simulink model "qpskrx_2022a"  (R2022a)
settings: Solver=FixedStepDiscrete  StartTime=0.0  StopTime=N*r/fs  RelTol=1e-3
values from neighbouring files (symbols this model uses):
  fs = oriFs*r    (= 750000000)    [LoadMat.m]    (also in test.m = 50000000; workspaceLoader.m = 75000000; workspaceLoader_fc32.m = 75000000; workspaceLoader_int16.m = 1500000000)
  rs = 75e6    (= 75000000)    [LoadMat.m]    (also in test.m = 37500000; workspaceLoader.m = 37500000; workspaceLoader_fc32.m = 37500000; workspaceLoader_int16.m)
libraries: commsync2 x2, commrfcorlib x1, dspsigops x1, commfilt2 x1
settings Model: FPTRunName=Active  Creator=The MathWorks, Inc.  LastModifiedBy=admin
settings SolverCC: AlgebraicLoopSolver=TrustRegion
settings DataIOCC: LimitDataPoints=on  SaveFormat=Structure  SaveOutput=off  SignalLogging=off  DSMLogging=off  SaveTime=off  ReturnWorkspaceOutputs=off
settings OptimizationCC: DefaultParameterBehavior=Inlined  ExpressionDepthLimit=2147483647  LocalBlockOutputs=off  ZeroExternalMemoryAtStartup=off  ZeroInternalMemoryAtStartup=off  InitFltsAndDblsToZero=on  LifeSpan=inf  SimCompilerOptimization=on
settings DebuggingCC: AlgebraicLoopMsg=error  UnderspecifiedInitializationDetection=Classic  MergeDetectMultiDrivingBlocksExec=none  SolverPrmCheckMsg=warning  SingleTaskRateTransMsg=error  ParameterPrecisionLossMsg=none  FcnCallInpInsideContextMsg=warning  UnconnectedInputMsg=warning  UnconnectedOutputMsg=warning  UnconnectedLineMsg=warning  AllowSymbolicDim=off  StateNameClashWarn=warning  SFUnexpectedBacktrackingDiag=warning  SFNoUnconditionalDefaultTransitionDiag=warning  SFExecutionAtInitializationDiag=none  ArithmeticOperatorsInVariantConditions=warning
settings HardwareCC: ProdBitPerPointer=32  ProdBitPerSizeT=32  ProdBitPerPtrDiffT=32  ProdLargestAtomicFloat=None  ProdIntDivRoundTo=Undefined  ProdEndianess=Unspecified  ProdWordSize=32  ProdLongLongMode=on  ProdHWDeviceType=32-bit Generic  TargetBitPerPointer=64  TargetBitPerSizeT=64  TargetBitPerPtrDiffT=64  TargetLongLongMode=on  TargetIntDivRoundTo=Zero  TargetEndianess=LittleEndian  TargetWordSize=64  TargetHWDeviceType=Generic->MATLAB Host Computer  ProdEqTarget=off
settings ModelReferenceCC: PropagateSignalLabelsOutOfModel=off
settings SFSimCC: SimUseLocalCustomCode=off  CustomCodeUndefinedFunction=UseInterfaceOnly  SimTargetLang=C++  GPUAcceleration=on  SimDLTargetLibrary=cudnn
settings RTWCC: RTWUseLocalCustomCode=off  TargetLang=C++  DLArmComputeVersion=19.05
settings RTWCC: CustomSourceCode=|
  | #include <stdio.h>
  | #include <stdlib.h>
settings CodeAppCC: StateflowObjectComments=on
settings GRTTargetCC: TargetLangStandard=C++11 (ISO)  CodeInterfacePackaging=C++ class
settings ConfigComp: CovMetricSettings=dw  CovSaveCumulativeToWorkspaceVar=on  CovSaveSingleToWorkspaceVar=on  CovExternalEMLEnable=off  CovSFcnEnable=off

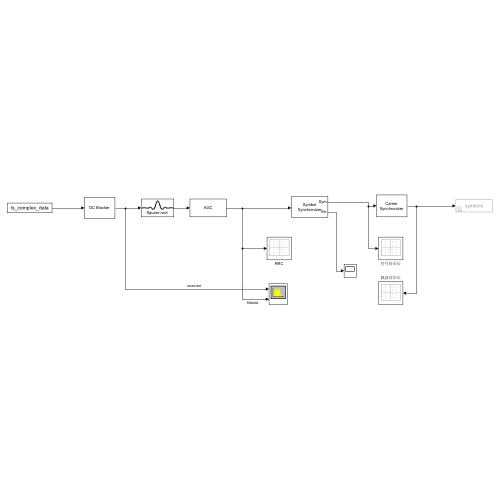
[thumbnail: Simulink's stored preview of the top-level diagram]
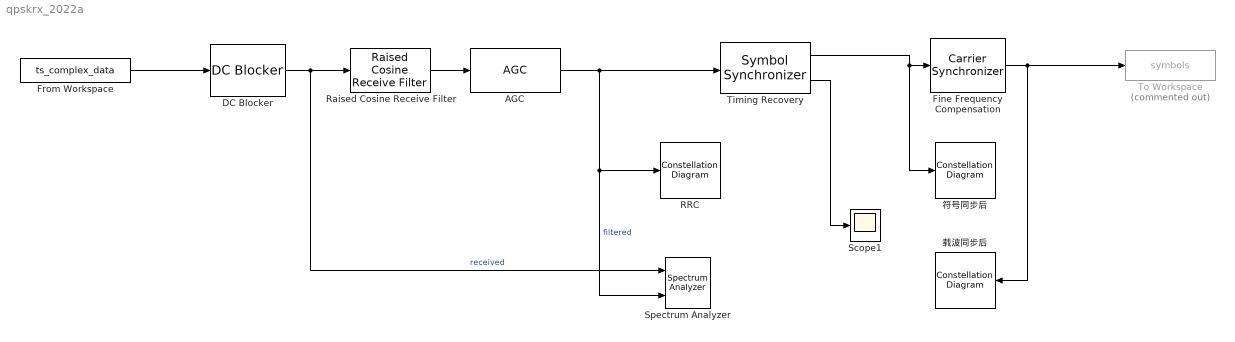
== system qpskrx_2022a ==
  AGC : commrfcorlib/AGC  LegacyMode=off  DetectorMethod=Rectifier  LoopMethod=Linear  UpdatePeriod=100  StepSize=0.1  AdaptationStepSize=0.1  DesiredOutputPower=0.6  AveragingLength=800  MaximumGain=30  MaxPowerGain=80  GainOutputPort=off  InputPowerOutputPort=off  SimulateUsing=Code generation
  DC Blocker : dspsigops/DC Blocker  Algorithm=IIR  NormalizedBandwidth=0.001  Length=8  Order=6  SimulateUsing=Code generation
  Fine Frequency Compensation : commsync2/Carrier Synchronizer  Modulation=QPSK  ModulationPhaseOffset=Auto  CustomPhaseOffset=0  SamplesPerSymbol=fs/rs  DampingFactor=1  NormalizedLoopBandwidth=0.01  EstimatedPhaseErrorOutputPort=off  SimulateUsing=Code generation
  From Workspace : FromWorkspace  VariableName=ts_complex_data  SampleTime=1/fs  OutputAfterFinalValue=Setting to zero
  RRC : ConstellationDiagram  WindowPosition=[46.000000,171.000000,600.000000,600.000000,]  Visible=on  ScopeFrameLocation=window  SymbolsToDisplaySource=Property  SymbolsToDisplay=200  XLimits=[-1.46,1.46]  YLimits=[-1.38,1.38]
  Raised Cosine Receive Filter : commfilt2/Raised Cosine Receive Filter  filtType=Square root  R=1/3  filtSpan=8  N=fs/rs  downFactor=1  downOffset=0  filterGain=1  RateOptions=Allow multirate processing  framing=Mute  checkCoeff=off  variableName=rcRxFilt  currentFiltSpan=10  D=5  inputOffset=0  sampMode=Mute  saveAsFlag=0  rateMode=Downsampling  checkGain=Normalized  launchFVT=on  roundingMode=Floor  overflowMode=off  coeffDataTypeStr=Inherit: Same word length as input  coeffMin=[]  coeffMax=[]  coeffLastDataTypeStr=Inherit: Same word length as input  accumDataTypeStr=Inherit: Same as product output  accumLastDataTypeStr=Inherit: Same as product output  outputDataTypeStr=Inherit: Same as accumulator  outputMin=[]  outputMax=[]  outputLastDataTypeStr=Inherit: Same as accumulator
  Scope1 : Scope
  Spectrum Analyzer : SpectrumAnalyzer  NumInputPorts=2  DefaultConfigurationName=spbscopes.SpectrumAnalyzerBlockCfg
  Timing Recovery : commsync2/Symbol Synchronizer  Modulation=PAM/PSK/QAM  TimingErrorDetector=Gardner (non-data-aided)  SamplesPerSymbol=fs/rs  DampingFactor=1  NormalizedLoopBandwidth=0.0002  DetectorGain=1  TimingErrorOutputPort=on  SimulateUsing=Code generation
  To Workspace : ToWorkspace  Commented=on  VariableName=symbols  SaveFormat=Timeseries  SampleTime=-1
      settings: Save2DSignal=2-D array (concatenate along first dimension)
  符号同步后 : ConstellationDiagram  WindowPosition=[638.000000,270.000000,600.000000,600.000000,]  Visible=on  ScopeFrameLocation=window  SymbolsToDisplaySource=Property  SymbolsToDisplay=200  XLimits=[-1.46,1.46]  YLimits=[-1.38,1.38]
  载波同步后 : ConstellationDiagram  WindowPosition=[1273.000000,217.000000,600.000000,600.000000,]  Visible=on  ScopeFrameLocation=window  SymbolsToDisplaySource=Property  SymbolsToDisplay=1000  XLimits=[-1.46,1.46]  YLimits=[-1.38,1.38]
  wires:
  Timing Recovery/1 -> 符号同步后/1, Fine Frequency Compensation/1
  DC Blocker/1 -> Spectrum Analyzer/1, Raised Cosine Receive Filter/1  "received"
  Raised Cosine Receive Filter/1 -> AGC/1
  AGC/1 -> Timing Recovery/1, RRC/1, Spectrum Analyzer/2  "filtered"
  From Workspace/1 -> DC Blocker/1
  Fine Frequency Compensation/1 -> To Workspace/1, 载波同步后/1
  Timing Recovery/2 -> Scope1/1
